simulink model "Ex6_1"  (Simulink 6.0)
settings: Solver=FixedStepDiscrete  StartTime=0.0  StopTime=Tstop  RelTol=1e-3
values from neighbouring files (symbols this model uses):
  Ampl = 0.85    [Ex6_1_Launch.m]
  dc = 1/7+0.001    (= 0.143857142857)    [Ex6_1_Launch.m]
  Kdc = 0    [Ex6_1_Launch.m]
  Ksine = 1    [Ex6_1_Launch.m]
  Nbit = 3    [Ex6_1_Launch.m]
  p_fft = 2^octaves    [Ex6_1_Launch.m]
  periods = 131    [Ex6_1_Launch.m]
settings Model: Creator=francomaloberti  LastModifiedBy=Cri  ExtModeAutoUpdateStatusClock=off
settings OptimizationCC: InlineInvariantSignals=off

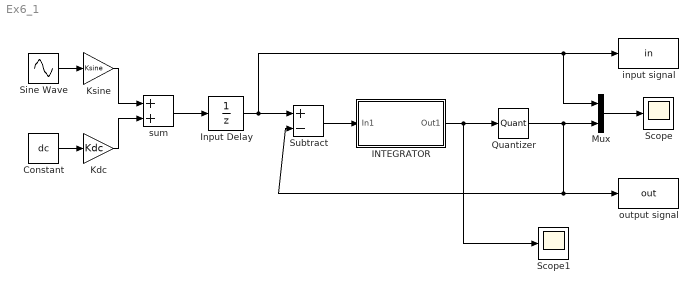
== system Ex6_1 ==
  Constant : Constant  Value=dc
  INTEGRATOR : Subsystem
      mask Display:
      | patch([0 20 0 0], [0 10 20 0],[0 1 0])
      | text(5,10,'\bf\int','texmode','on')
      | plot([0 20 0 0], [0 10 20 0])
  Input Delay : UnitDelay
  Kdc : Gain  Gain=Kdc
  Ksine : Gain  Gain=Ksine
  Mux : Mux  Inputs=2
  Quantizer : Quantizer  QuantizationInterval=1/2^Nbit
  Scope : Scope
      settings: TimeRange=200  YMin=-1.5  YMax=1.5
  Scope1 : Scope
      settings: TimeRange=500  YMin=-1.5  YMax=1.5
  Sine Wave : Sin  Amplitude=Ampl  Frequency=2*pi*periods/p_fft  Phase=01/21  SampleTime=0
  Subtract : Sum  Inputs=+-  OutScaling=2^-10
  input signal : ToWorkspace  VariableName=in  SampleTime=-1  SaveFormat=Array
  output signal : ToWorkspace  VariableName=out  SampleTime=-1  SaveFormat=Array
  sum : Sum  OutScaling=2^-10
  wires:
  Input Delay/1 -> Subtract/1, input signal/1, Mux/1
  Quantizer/1 -> Subtract/2, output signal/1, Mux/2
  Mux/1 -> Scope/1
  Constant/1 -> Kdc/1
  Sine Wave/1 -> Ksine/1
  Kdc/1 -> sum/2
  Ksine/1 -> sum/1
  sum/1 -> Input Delay/1
  Subtract/1 -> INTEGRATOR/1(In1)
  INTEGRATOR/1(Out1) -> Quantizer/1, Scope1/1

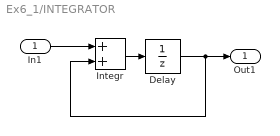
== system Ex6_1/INTEGRATOR ==
  In1 : Inport  Port=1  LatchInput=off
  Delay : UnitDelay
  Integr : Sum  OutScaling=2^-10
  Out1 : Outport
  wires:
  In1/1 -> Integr/1
  Integr/1 -> Delay/1
  Delay/1 -> Out1/1, Integr/2
